simulink model "pend_ss_d"  (Simulink 5.0)
settings: Solver=ode45  StartTime=0.0  StopTime=10.0  RelTol=1e-3
values from neighbouring files (symbols this model uses):
  K = place(A,B,P)    [pend_est.m]
  Ts = 0.01    [pend_est.m]
undefined symbols (not defined in the file or in its folder): a, b, c, d
settings Model: Creator=kannan  LastModifiedBy=kannanm  ExtModeAutoUpdateStatusClock=off

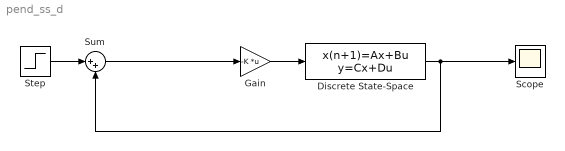
== system pend_ss_d ==
  Discrete State-Space : DiscreteStateSpace  A=a  B=b  C=c  D=d  X0=[0 0.1 0 0]  SampleTime=Ts
  Gain : Gain  Gain=-K  Multiplication=Matrix(K*u)  SaturateOnIntegerOverflow=on
  Scope : Scope
  Step : Step  After=0  SampleTime=Ts
  Sum : Sum  Inputs=|++  SaturateOnIntegerOverflow=on
  wires:
  Step/1 -> Sum/1
  Discrete State-Space/1 -> Scope/1, Sum/2
  Sum/1 -> Gain/1
  Gain/1 -> Discrete State-Space/1
